simulink model "SICARO"  (R2022b)
settings: Solver=ode23t  StartTime=0.0  StopTime=20  MaxStep=1e-3  RelTol=1e-3  AbsTol=1e-3
values from neighbouring files (symbols this model uses):
  air_rho = 1.225    [sicaro_inherited_params(stall).mat]
  battery_capacity = 22.8    [sicaro_inherited_params(stall).mat]
  CDO = 10.25    [sicaro_inherited_params(stall).mat]
  drag_linear = 0.002    [sicaro_inherited_params(stall).mat]
  drag_quad = 0.005    [sicaro_inherited_params(stall).mat]
  filtD_motor = 100    [sicaro_inherited_params(stall).mat]
  filtSpd_motor = 0.001    [sicaro_inherited_params(stall).mat]
  flap_radius = 0.05312    [sicaro_inherited_params(stall).mat]
  flap_surface_area = 0.025    [sicaro_inherited_params(stall).mat]
  kd_motor = 0    [sicaro_inherited_params(stall).mat]
  ki_motor = 0.00045    [sicaro_inherited_params(stall).mat]
  klinear = 0.03    [sicaro_inherited_params(stall).mat]
  kquad = 0.025    [sicaro_inherited_params(stall).mat]
  limit_motor = 0.25    [sicaro_inherited_params(stall).mat]
  monoco_mass = 160    [sicaro_inherited_params(stall).mat]
  monoco_prop =     [sicaro_inherited_params(stall).mat]
  monoco_radius = 0.61    [sicaro_inherited_params(stall).mat]
  monoco_wing =     [sicaro_inherited_params(stall).mat]
  monoco_wing_area = 0.239    [sicaro_inherited_params(stall).mat]
  waypoints = [-2 -2 0.14 -2 -2 6 0 0 6 2 0 6 ... (15 elements, 3x5)]    [sicaro_inherited_params(stall).mat]
undefined symbols (not defined in the file or in its folder): X, Y, Z
libraries: sm_lib x96, nesl_utility x38, slpidlib x20, fl_lib x12, sdl_lib x3, simulink x2, simulink_extras x1, batteryecm_lib x1, ee_lib x1
(part 4 of 7)

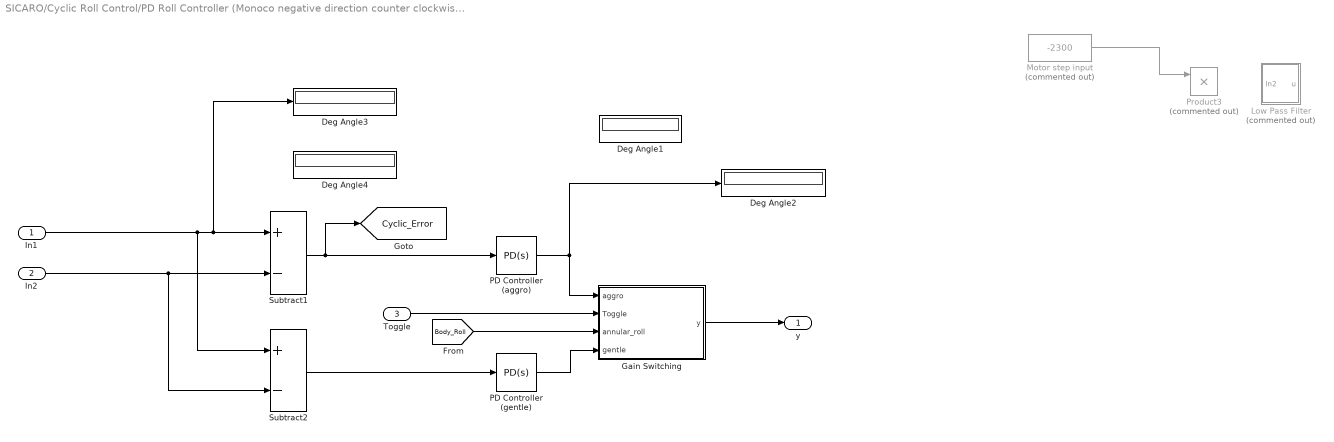
== system SICARO/Cyclic Roll Control/PD Roll Controller (Monoco negative direction counter clockwise) Front Motor ==
  In1 : Inport
  In2 : Inport  Port=2
  Toggle : Inport  Port=3
  Deg Angle{1..4} (4 alike) : Display
  Gain Switching : MATLAB Function  TreatAsAtomicUnit=on
  Low Pass Filter : Subsystem  Commented=on
  Motor step input : Constant  Commented=on  Value=-2300
  PD Controller (aggro) : slpidlib/PID Controller  Controller=PD  Form=Parallel  TimeDomain=Continuous-time  UseExternalTs=off  SampleTime=-1  IntegratorMethod=Forward Euler  FilterMethod=Forward Euler  ControllerParametersSource=internal  P=3  I=0.0  UseKiTs=off  D=2.7  N=filtD_motor  UseFilter=on  TunerSelectOption=Transfer Function Based (PID Tuner App)  InitialConditionSource=internal  InitialConditionForIntegrator=0  InitialConditionForFilter=0  DifferentiatorICPrevScaledInput=0  ExternalReset=none  TrackingMode=off  Kt=1  LimitOutput=off  SatLimitsSource=internal  UpperSaturationLimit=inf  LowerSaturationLimit=-inf  LinearizeAsGain=off  AntiWindupMode=none  Kb=1  LimitIntegrator=off  UpperIntegratorSaturationLimit=inf  LowerIntegratorSaturationLimit=-inf  POutMin=[]  POutMax=[]  IOutMin=[]  IOutMax=[]  DOutMin=[]  DOutMax=[]  NOutMin=[]  NOutMax=[]  SumOutMin=[]  SumOutMax=[]  SaturationOutMin=[]  SaturationOutMax=[]  PParamMin=[]  PParamMax=[]  IParamMin=[]  IParamMax=[]  DParamMin=[]  DParamMax=[]  NParamMin=[]  NParamMax=[]  KbParamMin=[]  KbParamMax=[]  KtParamMin=[]  KtParamMax=[]  KbOutMin=[]  KbOutMax=[]  KtOutMin=[]  KtOutMax=[]  IntegratorOutMin=[]  IntegratorOutMax=[]  FilterOutMin=[]  FilterOutMax=[]  SumI1OutMin=[]  SumI1OutMax=[]  SumI2OutMin=[]  SumI2OutMax=[]  SumI3OutMin=[]  SumI3OutMax=[]  SumI4OutMin=[]  SumI4OutMax=[]  SumDOutMin=[]  SumDOutMax=[]  DifferentiatorOutMin=[]  DifferentiatorOutMax=[]  FilterDiffOutCoefMin=[]  FilterDiffOutCoefMax=[]  ReciprocalOutMin=[]  ReciprocalOutMax=[]  SumDenOutMin=[]  SumDenOutMax=[]  SumNumOutMin=[]  SumNumOutMax=[]  DivideOutMin=[]  DivideOutMax=[]  UdiffTsProdOutMin=[]  UdiffTsProdOutMax=[]  NTsProdOutMin=[]  NTsProdOutMax=[]  UintegralTsProdOutMin=[]  UintegralTsProdOutMax=[]  UngainTsProdOutMin=[]  UngainTsProdOutMax=[]  ClampingZeroOutDataTypeStr=Inherit: Inherit via back propagation  ClampingZeroOutMin=[]  ClampingZeroOutMax=[]  FilterDenConstantOutDataTypeStr=Inherit: Inherit via back propagation  FilterDenConstantOutMin=[]  FilterDenConstantOutMax=[]  PCopyOutDataTypeStr=Inherit: Inherit via back propagation  PCopyOutMin=[]  PCopyOutMax=[]  NCopyOutDataTypeStr=Inherit: Inherit via back propagation  NCopyOutMin=[]  NCopyOutMax=[]  IntegratorContinuousStateAttributes=''  IntegratorStateMustResolveToSignalObject=off  IntegratorRTWStateStorageClass=Auto  FilterContinuousStateAttributes=''  FilterStateMustResolveToSignalObject=off  FilterRTWStateStorageClass=Auto  ParallelPVariant=InternalParameters  IdealPVariant=Disabled  IVariant=Disabled  DVariant=InternalParameters  IntegratorVariant=Disabled  SatVariant=Disabled  AWVariant=Disabled  PCopyVariant=Disabled  TRVariant=Disabled  FdbkBlocksVariant=Forward  IdealPFdbkVariant=Disabled  SatFdbkVariant=Disabled  DerivativeFilterVariant=ContFilter  NVariant=InternalParameters  NCopyVariant=Disabled  FilterICVariant=InternalICsFilter  IntegratorICVariant=Disabled  ExternalResetVariant=Disabled  TRSumVariant=Passthrough  SumFdbkVariant=Disabled  SumVariant=Sum_PD  TsampFilterVariant=InternalTs  TsampNgainVariant=Passthrough  TsampIntegralVariant=Disabled_SignalSpec  ExternalSaturationOutDataTypeStr=Inherit: Same as second input
      settings: LibrarySourceBlock=simulink/Discrete/Discrete PID Controller
  PD Controller (gentle) : slpidlib/PID Controller  Controller=PD  Form=Parallel  TimeDomain=Continuous-time  UseExternalTs=off  SampleTime=-1  IntegratorMethod=Forward Euler  FilterMethod=Forward Euler  ControllerParametersSource=internal  P=1.5  I=0.0  UseKiTs=off  D=1.35  N=filtD_motor  UseFilter=on  TunerSelectOption=Transfer Function Based (PID Tuner App)  InitialConditionSource=internal  InitialConditionForIntegrator=0  InitialConditionForFilter=0  DifferentiatorICPrevScaledInput=0  ExternalReset=none  TrackingMode=off  Kt=1  LimitOutput=off  SatLimitsSource=internal  UpperSaturationLimit=inf  LowerSaturationLimit=-inf  LinearizeAsGain=off  AntiWindupMode=none  Kb=1  LimitIntegrator=off  UpperIntegratorSaturationLimit=inf  LowerIntegratorSaturationLimit=-inf  POutMin=[]  POutMax=[]  IOutMin=[]  IOutMax=[]  DOutMin=[]  DOutMax=[]  NOutMin=[]  NOutMax=[]  SumOutMin=[]  SumOutMax=[]  SaturationOutMin=[]  SaturationOutMax=[]  PParamMin=[]  PParamMax=[]  IParamMin=[]  IParamMax=[]  DParamMin=[]  DParamMax=[]  NParamMin=[]  NParamMax=[]  KbParamMin=[]  KbParamMax=[]  KtParamMin=[]  KtParamMax=[]  KbOutMin=[]  KbOutMax=[]  KtOutMin=[]  KtOutMax=[]  IntegratorOutMin=[]  IntegratorOutMax=[]  FilterOutMin=[]  FilterOutMax=[]  SumI1OutMin=[]  SumI1OutMax=[]  SumI2OutMin=[]  SumI2OutMax=[]  SumI3OutMin=[]  SumI3OutMax=[]  SumI4OutMin=[]  SumI4OutMax=[]  SumDOutMin=[]  SumDOutMax=[]  DifferentiatorOutMin=[]  DifferentiatorOutMax=[]  FilterDiffOutCoefMin=[]  FilterDiffOutCoefMax=[]  ReciprocalOutMin=[]  ReciprocalOutMax=[]  SumDenOutMin=[]  SumDenOutMax=[]  SumNumOutMin=[]  SumNumOutMax=[]  DivideOutMin=[]  DivideOutMax=[]  UdiffTsProdOutMin=[]  UdiffTsProdOutMax=[]  NTsProdOutMin=[]  NTsProdOutMax=[]  UintegralTsProdOutMin=[]  UintegralTsProdOutMax=[]  UngainTsProdOutMin=[]  UngainTsProdOutMax=[]  ClampingZeroOutDataTypeStr=Inherit: Inherit via back propagation  ClampingZeroOutMin=[]  ClampingZeroOutMax=[]  FilterDenConstantOutDataTypeStr=Inherit: Inherit via back propagation  FilterDenConstantOutMin=[]  FilterDenConstantOutMax=[]  PCopyOutDataTypeStr=Inherit: Inherit via back propagation  PCopyOutMin=[]  PCopyOutMax=[]  NCopyOutDataTypeStr=Inherit: Inherit via back propagation  NCopyOutMin=[]  NCopyOutMax=[]  IntegratorContinuousStateAttributes=''  IntegratorStateMustResolveToSignalObject=off  IntegratorRTWStateStorageClass=Auto  FilterContinuousStateAttributes=''  FilterStateMustResolveToSignalObject=off  FilterRTWStateStorageClass=Auto  ParallelPVariant=InternalParameters  IdealPVariant=Disabled  IVariant=Disabled  DVariant=InternalParameters  IntegratorVariant=Disabled  SatVariant=Disabled  AWVariant=Disabled  PCopyVariant=Disabled  TRVariant=Disabled  FdbkBlocksVariant=Forward  IdealPFdbkVariant=Disabled  SatFdbkVariant=Disabled  DerivativeFilterVariant=ContFilter  NVariant=InternalParameters  NCopyVariant=Disabled  FilterICVariant=InternalICsFilter  IntegratorICVariant=Disabled  ExternalResetVariant=Disabled  TRSumVariant=Passthrough  SumFdbkVariant=Disabled  SumVariant=Sum_PD  TsampFilterVariant=InternalTs  TsampNgainVariant=Passthrough  TsampIntegralVariant=Disabled_SignalSpec  ExternalSaturationOutDataTypeStr=Inherit: Same as second input
      settings: LibrarySourceBlock=simulink/Discrete/Discrete PID Controller
  Product3 : Product  Commented=on
  Subtract1 : Sum  Inputs=+-
  Subtract2 : Sum  Inputs=+-
  y : Outport
  tag scope: Cyclic_Error=global
  wires:
  Motor step input/1 -> Product3/1
  PD Controller (aggro)/1 -> Deg Angle2/1, Gain Switching/1(aggro)
  Subtract1/1 -> PD Controller (aggro)/1, [Cyclic_Error]
  Subtract2/1 -> PD Controller (gentle)/1
  Gain Switching/1(y) -> y/1
  PD Controller (gentle)/1 -> Gain Switching/4(gentle)
  Toggle/1 -> Gain Switching/2(Toggle)
  [Body_Roll] -> Gain Switching/3(annular_roll)
  In1/1 -> Subtract1/1, Deg Angle3/1, Subtract2/1
  In2/1 -> Subtract2/2, Subtract1/2

== system SICARO/Cyclic Roll Control/PD Roll Controller (Monoco positve direction clockwise) ==
  In2 : Inport
  In1 : Inport  Port=2
  Discrete PD Controller : slpidlib/PID Controller  Controller=PD  Form=Parallel  TimeDomain=Continuous-time  UseExternalTs=off  SampleTime=-1  IntegratorMethod=Forward Euler  FilterMethod=Forward Euler  ControllerParametersSource=internal  P=5.35  I=0.0  UseKiTs=off  D=1.25  N=filtD_motor  UseFilter=on  TunerSelectOption=Transfer Function Based (PID Tuner App)  InitialConditionSource=internal  InitialConditionForIntegrator=0  InitialConditionForFilter=0  DifferentiatorICPrevScaledInput=0  ExternalReset=none  TrackingMode=off  Kt=1  LimitOutput=off  SatLimitsSource=internal  UpperSaturationLimit=inf  LowerSaturationLimit=-inf  LinearizeAsGain=off  AntiWindupMode=none  Kb=1  LimitIntegrator=off  UpperIntegratorSaturationLimit=inf  LowerIntegratorSaturationLimit=-inf  POutMin=[]  POutMax=[]  IOutMin=[]  IOutMax=[]  DOutMin=[]  DOutMax=[]  NOutMin=[]  NOutMax=[]  SumOutMin=[]  SumOutMax=[]  SaturationOutMin=[]  SaturationOutMax=[]  PParamMin=[]  PParamMax=[]  IParamMin=[]  IParamMax=[]  DParamMin=[]  DParamMax=[]  NParamMin=[]  NParamMax=[]  KbParamMin=[]  KbParamMax=[]  KtParamMin=[]  KtParamMax=[]  KbOutMin=[]  KbOutMax=[]  KtOutMin=[]  KtOutMax=[]  IntegratorOutMin=[]  IntegratorOutMax=[]  FilterOutMin=[]  FilterOutMax=[]  SumI1OutMin=[]  SumI1OutMax=[]  SumI2OutMin=[]  SumI2OutMax=[]  SumI3OutMin=[]  SumI3OutMax=[]  SumI4OutMin=[]  SumI4OutMax=[]  SumDOutMin=[]  SumDOutMax=[]  DifferentiatorOutMin=[]  DifferentiatorOutMax=[]  FilterDiffOutCoefMin=[]  FilterDiffOutCoefMax=[]  ReciprocalOutMin=[]  ReciprocalOutMax=[]  SumDenOutMin=[]  SumDenOutMax=[]  SumNumOutMin=[]  SumNumOutMax=[]  DivideOutMin=[]  DivideOutMax=[]  UdiffTsProdOutMin=[]  UdiffTsProdOutMax=[]  NTsProdOutMin=[]  NTsProdOutMax=[]  UintegralTsProdOutMin=[]  UintegralTsProdOutMax=[]  UngainTsProdOutMin=[]  UngainTsProdOutMax=[]  ClampingZeroOutDataTypeStr=Inherit: Inherit via back propagation  ClampingZeroOutMin=[]  ClampingZeroOutMax=[]  FilterDenConstantOutDataTypeStr=Inherit: Inherit via back propagation  FilterDenConstantOutMin=[]  FilterDenConstantOutMax=[]  PCopyOutDataTypeStr=Inherit: Inherit via back propagation  PCopyOutMin=[]  PCopyOutMax=[]  NCopyOutDataTypeStr=Inherit: Inherit via back propagation  NCopyOutMin=[]  NCopyOutMax=[]  IntegratorContinuousStateAttributes=''  IntegratorStateMustResolveToSignalObject=off  IntegratorRTWStateStorageClass=Auto  FilterContinuousStateAttributes=''  FilterStateMustResolveToSignalObject=off  FilterRTWStateStorageClass=Auto  ParallelPVariant=InternalParameters  IdealPVariant=Disabled  IVariant=Disabled  DVariant=InternalParameters  IntegratorVariant=Disabled  SatVariant=Disabled  AWVariant=Disabled  PCopyVariant=Disabled  TRVariant=Disabled  FdbkBlocksVariant=Forward  IdealPFdbkVariant=Disabled  SatFdbkVariant=Disabled  DerivativeFilterVariant=ContFilter  NVariant=InternalParameters  NCopyVariant=Disabled  FilterICVariant=InternalICsFilter  IntegratorICVariant=Disabled  ExternalResetVariant=Disabled  TRSumVariant=Passthrough  SumFdbkVariant=Disabled  SumVariant=Sum_PD  TsampFilterVariant=InternalTs  TsampNgainVariant=Passthrough  TsampIntegralVariant=Disabled_SignalSpec  ExternalSaturationOutDataTypeStr=Inherit: Same as second input
      settings: LibrarySourceBlock=simulink/Discrete/Discrete PID Controller
  Offset : Subsystem
  Subtract1 : Sum  Inputs=+-
  Out1 : Outport
  wires:
  In2/1 -> Offset/1(In2)
  Offset/1(Out1) -> Subtract1/1
  Subtract1/1 -> Discrete PD Controller/1
  In1/1 -> Subtract1/2
  Discrete PD Controller/1 -> Out1/1

== system SICARO/Misc Functions/Control ==
  ref : Inport
  meas : Inport  Port=2
  Add : Sum  Inputs=+-
  Control : slpidlib/PID Controller  Controller=PID  Form=Parallel  TimeDomain=Continuous-time  UseExternalTs=off  SampleTime=-1  IntegratorMethod=Forward Euler  FilterMethod=Forward Euler  ControllerParametersSource=internal  P=2  I=ki_motor  UseKiTs=off  D=kd_motor  N=filtD_motor  UseFilter=on  TunerSelectOption=Transfer Function Based (PID Tuner App)  ZeroCross=off  InitialConditionSource=internal  InitialConditionForIntegrator=0  InitialConditionForFilter=0  DifferentiatorICPrevScaledInput=0  ExternalReset=none  TrackingMode=off  Kt=1  LimitOutput=on  SatLimitsSource=internal  UpperSaturationLimit=limit_motor  LowerSaturationLimit=-limit_motor  LinearizeAsGain=on  AntiWindupMode=clamping  Kb=1  LimitIntegrator=off  UpperIntegratorSaturationLimit=inf  LowerIntegratorSaturationLimit=-inf  POutMin=[]  POutMax=[]  IOutMin=[]  IOutMax=[]  DOutMin=[]  DOutMax=[]  NOutMin=[]  NOutMax=[]  SumOutMin=[]  SumOutMax=[]  SaturationOutMin=[]  SaturationOutMax=[]  PParamMin=[]  PParamMax=[]  IParamMin=[]  IParamMax=[]  DParamMin=[]  DParamMax=[]  NParamMin=[]  NParamMax=[]  KbParamMin=[]  KbParamMax=[]  KtParamMin=[]  KtParamMax=[]  KbOutMin=[]  KbOutMax=[]  KtOutMin=[]  KtOutMax=[]  IntegratorOutMin=[]  IntegratorOutMax=[]  FilterOutMin=[]  FilterOutMax=[]  SumI1OutMin=[]  SumI1OutMax=[]  SumI2OutMin=[]  SumI2OutMax=[]  SumI3OutMin=[]  SumI3OutMax=[]  SumI4OutMin=[]  SumI4OutMax=[]  SumDOutMin=[]  SumDOutMax=[]  DifferentiatorOutMin=[]  DifferentiatorOutMax=[]  FilterDiffOutCoefMin=[]  FilterDiffOutCoefMax=[]  ReciprocalOutMin=[]  ReciprocalOutMax=[]  SumDenOutMin=[]  SumDenOutMax=[]  SumNumOutMin=[]  SumNumOutMax=[]  DivideOutMin=[]  DivideOutMax=[]  UdiffTsProdOutMin=[]  UdiffTsProdOutMax=[]  NTsProdOutMin=[]  NTsProdOutMax=[]  UintegralTsProdOutMin=[]  UintegralTsProdOutMax=[]  UngainTsProdOutMin=[]  UngainTsProdOutMax=[]  ClampingZeroOutDataTypeStr=Inherit: Inherit via back propagation  ClampingZeroOutMin=[]  ClampingZeroOutMax=[]  FilterDenConstantOutDataTypeStr=Inherit: Inherit via back propagation  FilterDenConstantOutMin=[]  FilterDenConstantOutMax=[]  PCopyOutDataTypeStr=Inherit: Inherit via back propagation  PCopyOutMin=[]  PCopyOutMax=[]  NCopyOutDataTypeStr=Inherit: Inherit via back propagation  NCopyOutMin=[]  NCopyOutMax=[]  IntegratorContinuousStateAttributes=''  IntegratorStateMustResolveToSignalObject=off  IntegratorRTWStateStorageClass=Auto  FilterContinuousStateAttributes=''  FilterStateMustResolveToSignalObject=off  FilterRTWStateStorageClass=Auto  ParallelPVariant=InternalParameters  IdealPVariant=Disabled  IVariant=InternalParameters  DVariant=InternalParameters  IntegratorVariant=Continuous  SatVariant=Enabled  AWVariant=ContClampingParallel  PCopyVariant=Disabled  TRVariant=Disabled  FdbkBlocksVariant=Forward  IdealPFdbkVariant=Disabled  SatFdbkVariant=Disabled  DerivativeFilterVariant=ContFilter  NVariant=InternalParameters  NCopyVariant=Disabled  FilterICVariant=InternalICsFilter  IntegratorICVariant=InternalICs  ExternalResetVariant=Disabled  TRSumVariant=Passthrough  SumFdbkVariant=Disabled  SumVariant=Sum_PID  TsampFilterVariant=InternalTs  TsampNgainVariant=Passthrough  TsampIntegralVariant=Passthrough  ExternalSaturationOutDataTypeStr=Inherit: Same as second input
  Mux : Mux  Inputs=2
  Scope : Scope  NumInputPorts=3
  Transfer Fcn1 : TransferFcn  Denominator=[filtSpd_motor 1]  ParameterTunability=Optimized
  torque : Outport
  wires:
  Control/1 -> torque/1, Scope/3  "torque"
  ref/1 -> Add/1, Mux/1
  Add/1 -> Scope/2, Control/1  "error"
  Mux/1 -> Scope/1
  Transfer Fcn1/1 -> Mux/2, Add/2
  meas/1 -> Transfer Fcn1/1

== system SICARO/Misc Functions/Thrust and Drag ==
  PS-Simulink Converter : nesl_utility/PS-Simulink Converter  PhysicalDomain=network_engine_domain  SubClassName=ps_output  LeftPortType=input  RightPortType=output  PseudoPeriodic=off  Frequencies=[]  VectorFormat=1-D array  Unit=inherit  AffineConversion=off
  PS-Simulink Converter1 : nesl_utility/PS-Simulink Converter  PhysicalDomain=network_engine_domain  SubClassName=ps_output  LeftPortType=input  RightPortType=output  PseudoPeriodic=off  Frequencies=[]  VectorFormat=inherit  Unit=inherit  AffineConversion=off
  PS-Simulink Converter2 : nesl_utility/PS-Simulink Converter  PhysicalDomain=network_engine_domain  SubClassName=ps_output  LeftPortType=input  RightPortType=output  PseudoPeriodic=off  Frequencies=[]  VectorFormat=inherit  Unit=inherit  AffineConversion=off
  PS-Simulink Converter3 : nesl_utility/PS-Simulink Converter  PhysicalDomain=network_engine_domain  SubClassName=ps_output  LeftPortType=input  RightPortType=output  PseudoPeriodic=off  Frequencies=[]  VectorFormat=1-D array  Unit=inherit  AffineConversion=off
  Prop Force Thrust and Drag : sm_lib/Forces and Torques/External Force and Torque  Commented=on  ForceResolutionFrame=AttachedFrame  EnableForceX=off  EnableForceY=off  EnableForceZ=on  EnableForce=off  TorqueResolutionFrame=AttachedFrame  EnableTorqueX=off  EnableTorqueY=off  EnableTorqueZ=on  EnableTorque=off
  Speed of flow through prop : fl_lib/Physical Signals/Sources/PS Constant  constant=0.1 m/s
  Thrust and Drag : Subsystem  AncestorBlock=quadcopter_library/Propeller/Thrust and Drag
      settings: LibrarySourceBlock=quadcopter_library/Propeller/Thrust and Drag
      mask Display: image('C:\Users\emman\Monocopter_Frame\three-bladed-boat-propeller.jpg'); % Use "Edit Image" on toolstrip to change.
  Transform Sensor : sm_lib/Frames and Transforms/Transform Sensor  MeasurementFrame=Follower  SenseAngle=off  SenseAxis=off  SenseQ=off  SenseR=off  SenseRotationSequence=off  RotationSequence=XYX  SenseOmegaX=off  SenseOmegaY=off  SenseOmegaZ=on  SenseQDot=off  SenseRDot=off  SenseAlphaX=off  SenseAlphaY=off  SenseAlphaZ=off  SenseQDDot=off  SenseRDDot=off  SenseX=off  SenseY=off  SenseZ=off  SenseRad=off  SenseAzim=off  SenseDist=off  SenseInc=off  SenseXDot=off  SenseYDot=off  SenseZDot=off  SenseRadDot=off  SenseAzimDot=off  SenseDistDot=off  SenseIncDot=off  SenseXDDot=off  SenseYDDot=off  SenseZDDot=off  SenseRadDDot=off  SenseAzimDDot=off  SenseDistDDot=off  SenseIncDDot=off
  World Frame : sm_lib/Frames and Transforms/World Frame
  F : PMIOPort  Side=Left
  prop thrust : Outport
  prop torque : Outport  Port=2
  tag scope: Flow_Speed=global, Prop_Speed=global
  wires:
  PS-Simulink Converter/1 -> prop thrust/1
  PS-Simulink Converter1/1 -> [Prop_Speed]
  PS-Simulink Converter2/1 -> [Flow_Speed]
  PS-Simulink Converter3/1 -> prop torque/1
  connections:
  Thrust and Drag/LConn2 -- PS-Simulink Converter2/LConn1 -- Speed of flow through prop/RConn1
  Prop Force Thrust and Drag/RConn1 -- Transform Sensor/RConn1 -- F/RConn1
  Transform Sensor/LConn1 -- World Frame/RConn1
  Thrust and Drag/RConn2 -- PS-Simulink Converter/LConn1 -- Prop Force Thrust and Drag/LConn1
  Transform Sensor/RConn2 -- PS-Simulink Converter1/LConn1 -- Thrust and Drag/LConn1
  Prop Force Thrust and Drag/LConn2 -- PS-Simulink Converter3/LConn1 -- Thrust and Drag/RConn1

== system SICARO/Monowing/Collective Control ==
  Clock : Clock
  Collective (Anhedral) : MATLAB Function  TreatAsAtomicUnit=on
  Collective (Dihedral) : MATLAB Function  TreatAsAtomicUnit=on
  Collective Mode Switcher : MATLAB Function  TreatAsAtomicUnit=on
  Torque result : Display
  Dihedral : Outport
  Anhedral : Outport  Port=2
  wires:
  Collective Mode Switcher/1(dihedral) -> Collective (Dihedral)/2(Toggle)
  Collective (Anhedral)/1(output) -> Anhedral/1
  [Torque_from_motor_negative] -> Collective (Dihedral)/1(Torque_negative)
  Collective (Dihedral)/1(output) -> Torque result/1, Dihedral/1
  [Mode_Selection] -> Collective Mode Switcher/2(Mode)
  Clock/1 -> Collective Mode Switcher/1(Time)
  [Torque_from_motor_negative] -> Collective (Anhedral)/1(Torque_negative)

== system SICARO/Monowing/Drag State ==
  drag : Inport
  Clock3 : Clock
  Drag filter : MATLAB Function  TreatAsAtomicUnit=on
  drag_upper : Outport
  drag_lower : Outport  Port=2
  wires:
  [Mode_Selection] -> Drag filter/3(Mode)
  Drag filter/2(drag_lower) -> drag_lower/1
  Clock3/1 -> Drag filter/2(Time)
  drag/1 -> Drag filter/1(drag)
  Drag filter/1(drag_upper) -> drag_upper/1

== system SICARO/Monowing/Drag moment ==
  Drag Moment (X & Y) : MATLAB Function  TreatAsAtomicUnit=on
  Simulink-PS Converter2 : nesl_utility/Simulink-PS Converter  PhysicalDomain=network_engine_domain  SubClassName=ps_input  LeftPortType=input  RightPortType=output  PseudoPeriodic=off  Frequencies=[]  NoiseDistribution=none  NoiseParameters=[]  Unit=1  AffineConversion=off  FilteringAndDerivatives=provide  SimscapeFilterOrder=1  InputFilterTimeConstant=0.001  UdotUserProvided=0
  Simulink-PS Converter3 : nesl_utility/Simulink-PS Converter  PhysicalDomain=network_engine_domain  SubClassName=ps_input  LeftPortType=input  RightPortType=output  PseudoPeriodic=off  Frequencies=[]  NoiseDistribution=none  NoiseParameters=[]  Unit=1  AffineConversion=off  FilteringAndDerivatives=provide  SimscapeFilterOrder=1  InputFilterTimeConstant=0.001  UdotUserProvided=0
  Unit Delay : UnitDelay  SampleTime=10  HasFrameUpgradeWarning=on
  Unit Delay1 : UnitDelay  SampleTime=10  HasFrameUpgradeWarning=on
  drag moment abt y axis : Display
  output x : PMIOPort  Side=Right
  output y : PMIOPort  Port=2  Side=Right
  wires:
  Drag Moment (X & Y)/1(drag_moment_abt_y) -> drag moment abt y axis/1, Simulink-PS Converter2/1
  [angular_v_abt_y] -> Unit Delay/1
  Drag Moment (X & Y)/2(drag_moment_abt_x) -> Simulink-PS Converter3/1
  Unit Delay/1 -> Drag Moment (X & Y)/1(y)
  Unit Delay1/1 -> Drag Moment (X & Y)/2(x)
  [angular_v_abt_x] -> Unit Delay1/1
  [Azimuth] -> Drag Moment (X & Y)/3(azimuth)
  connections:
  Simulink-PS Converter2/RConn1 -- output y/RConn1
  Simulink-PS Converter3/RConn1 -- output x/RConn1

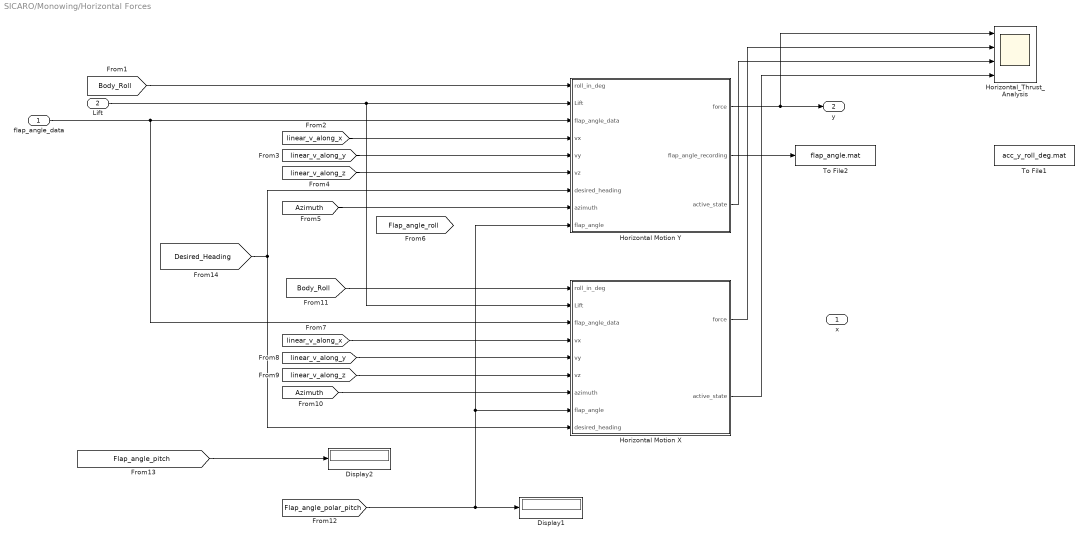
== system SICARO/Monowing/Horizontal Forces ==
  flap_angle_data : Inport
  Lift : Inport  Port=2
  Display1 : Display
  Display2 : Display
  Horizontal Motion X : MATLAB Function  TreatAsAtomicUnit=on
  Horizontal Motion Y : MATLAB Function  TreatAsAtomicUnit=on
  Horizontal_Thrust_Analysis : Scope  NumInputPorts=4
  To File1 : ToFile  Filename=acc_y_roll_deg.mat  MatrixName=acc_y
  To File2 : ToFile  Filename=flap_angle.mat  MatrixName=flap
  x : Outport
  y : Outport  Port=2
  wires:
  [linear_v_along_x] -> Horizontal Motion Y/4(vx)
  Horizontal Motion Y/2(flap_angle_recording) -> To File2/1
  [Body_Roll] -> Horizontal Motion Y/1(roll_in_deg)
  flap_angle_data/1 -> Horizontal Motion X/3(flap_angle_data), Horizontal Motion Y/3(flap_angle_data)
  Horizontal Motion Y/1(force) -> y/1, Horizontal_Thrust_Analysis/1
  [linear_v_along_z] -> Horizontal Motion Y/6(vz)
  [linear_v_along_y] -> Horizontal Motion Y/5(vy)
  Lift/1 -> Horizontal Motion Y/2(Lift), Horizontal Motion X/2(Lift)
  [Azimuth] -> Horizontal Motion Y/8(azimuth)
  [linear_v_along_y] -> Horizontal Motion X/5(vy)
  [linear_v_along_x] -> Horizontal Motion X/4(vx)
  [linear_v_along_z] -> Horizontal Motion X/6(vz)
  [Azimuth] -> Horizontal Motion X/7(azimuth)
  [Body_Roll] -> Horizontal Motion X/1(roll_in_deg)
  [Desired_Heading] -> Horizontal Motion X/9(desired_heading), Horizontal Motion Y/7(desired_heading)
  [Flap_angle_polar_pitch] -> Horizontal Motion Y/9(flap_angle), Horizontal Motion X/8(flap_angle), Display1/1
  [Flap_angle_pitch] -> Display2/1
  Horizontal Motion X/1(force) -> Horizontal_Thrust_Analysis/2
  Horizontal Motion Y/3(active_state) -> Horizontal_Thrust_Analysis/3
  Horizontal Motion X/2(active_state) -> Horizontal_Thrust_Analysis/4

== system SICARO/Monowing/Incremental Lift 4 mid ==
  In1 : Inport
  1/8 : Constant  Value=1/6
  Air_Rho : Constant  Value=air_rho
  Blade Chord : Constant  Value=monoco_wing_area/monoco_radius
  Conversion to Hz (Rotational Freq) : Constant  Value=0.1591549
  Lift Coeff : Constant  Value=monoco_wing.CL
  Math Function : Math  Operator=square
  Math Function1 : Math  Operator=pow
  Monoco Radius : Constant  Value=monoco_radius-0.176-0.201
  Product : Product  Inputs=6
  Product1 : Product
  Radius pow : Constant  Value=3
  Out1 : Outport
  wires:
  Lift Coeff/1 -> Product/6
  Math Function1/1 -> Product/4
  Product/1 -> Out1/1
  Conversion to Hz (Rotational Freq)/1 -> Product1/2
  Air_Rho/1 -> Product/3
  Product1/1 -> Math Function/1
  Radius pow/1 -> Math Function1/2
  Math Function/1 -> Product/1
  Blade Chord/1 -> Product/5
  In1/1 -> Product1/1
  Monoco Radius/1 -> Math Function1/1
  1/8/1 -> Product/2

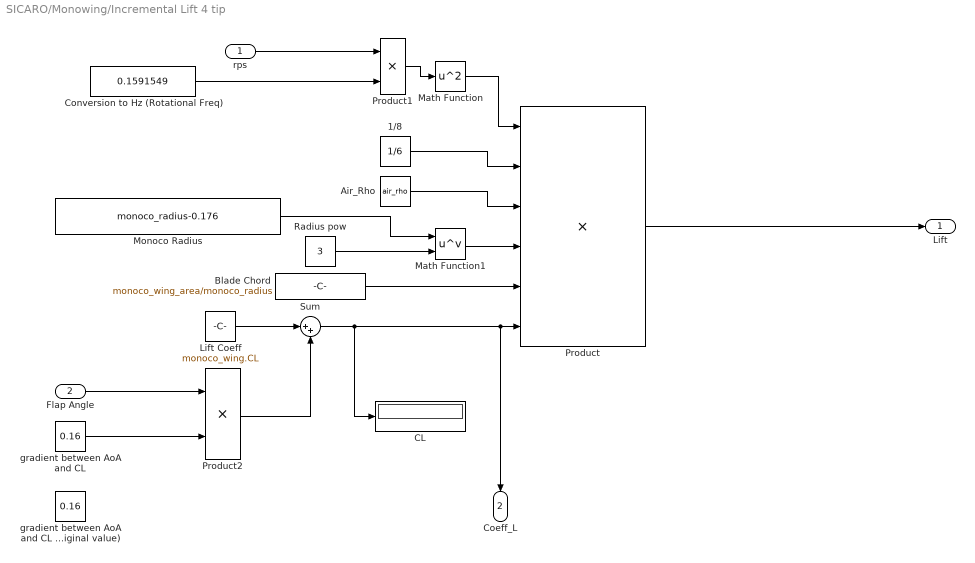
== system SICARO/Monowing/Incremental Lift 4 tip ==
  rps : Inport
  Flap Angle : Inport  Port=2
  1/8 : Constant  Value=1/6
  Air_Rho : Constant  Value=air_rho
  Blade Chord : Constant  Value=monoco_wing_area/monoco_radius
  CL : Display
  Conversion to Hz (Rotational Freq) : Constant  Value=0.1591549
  Lift Coeff : Constant  Value=monoco_wing.CL
  Math Function : Math  Operator=square
  Math Function1 : Math  Operator=pow
  Monoco Radius : Constant  Value=monoco_radius-0.176
  Product : Product  Inputs=6
  Product1 : Product
  Product2 : Product
  Radius pow : Constant  Value=3
  Sum : Sum  Inputs=|++
  gradient between AoA and CL : Constant  Value=0.16
  gradient between AoA and CL (original value) : Constant  Value=0.16
  Lift : Outport
  Coeff_L : Outport  Port=2
  wires:
  Math Function1/1 -> Product/4
  Product/1 -> Lift/1
  Air_Rho/1 -> Product/3
  Product1/1 -> Math Function/1
  Radius pow/1 -> Math Function1/2
  Math Function/1 -> Product/1
  Blade Chord/1 -> Product/5
  rps/1 -> Product1/1
  Monoco Radius/1 -> Math Function1/1
  1/8/1 -> Product/2
  Conversion to Hz (Rotational Freq)/1 -> Product1/2
  Lift Coeff/1 -> Sum/1
  Flap Angle/1 -> Product2/1
  Product2/1 -> Sum/2
  gradient between AoA and CL/1 -> Product2/2
  Sum/1 -> CL/1, Product/6, Coeff_L/1
